simulink model "test"  (R2024a)
settings: Solver=VariableStepAuto  StartTime=0.0  StopTime=1000  RelTol=1e-3
undefined symbols (not defined in the file or in its folder): x
libraries: simulink x2
settings Model: Creator=b_ant  LastModifiedBy=b_ant

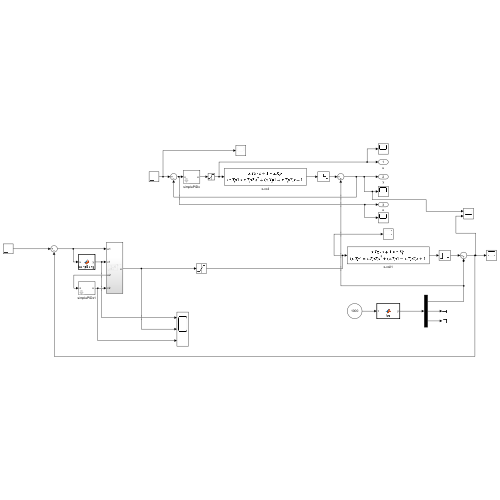
[thumbnail: Simulink's stored preview of the top-level diagram]
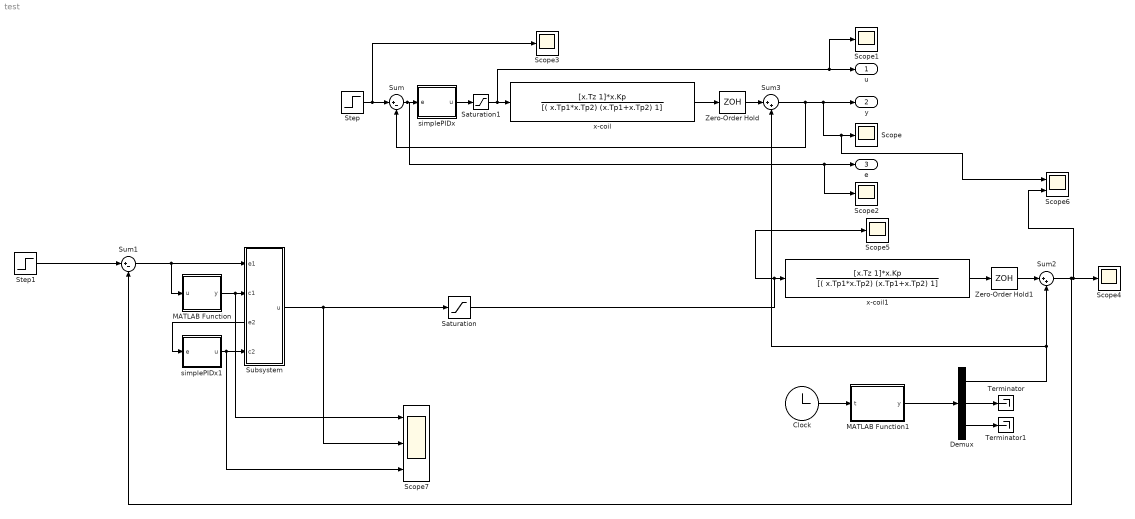
== system test ==
  Clock : Clock
  Demux : Demux  Outputs=3
  MATLAB Function : MATLAB Function  TreatAsAtomicUnit=on
  MATLAB Function1 : MATLAB Function  TreatAsAtomicUnit=on
  Saturation : Saturate  UpperLimit=15  LowerLimit=-15
  Saturation1 : Saturate  UpperLimit=15  LowerLimit=-15
  Scope{,1..5} (6 alike) : Scope
  Scope6 : Scope  NumInputPorts=2
  Scope7 : Scope  NumInputPorts=3
  Step : Step  Time=0.0001  SampleTime=0
  Step1 : Step  Time=0.0001  SampleTime=0
  Subsystem : Subsystem
      settings: PortSchema="{\"entries\":[{\"content\":{\"sides\":[{\"content\":{\"connectorIds\":[\"In1\",\"In2\",\"Out2\",\"In3\"]},\"type\":\"ConnectorPlacement.EquallySpacedRectSide\",\"uuid\":\"7068f7a8-39a5-4b81-9242-0ff684ad2d52\"},{\"content\":{\"connectorIds\":[\"Out1\"],\"side\":\"RIGHT\"},\"type\":\"ConnectorPlacement.EquallySpacedRectSide\",\"uuid\":\"6f619d2f-5996-4772-917a-a91f12c99af0\"},{\"content\":{\"side\":\"TOP\"},\"type\":\"ConnectorPlacement.EquallySpacedRectSide\",\"uuid\":\"a18f3392-cfd4-4b10-bccf-639e40fe0ff5\"}]},\"type\":\"ConnectorPlacement.EquallySpacedConnector\",\"uuid\":\"3030bedd-17ea-4c41-8905-7d24d55e9816\"}],\"packageUris\":[\"http://schema.mathworks.com/mf0/Connector/R2020b\"],\"version\":\"1.0\"}"
  Sum : Sum  Inputs=|+-
  Sum1 : Sum  Inputs=|+-
  Sum2 : Sum  Inputs=|++
  Sum3 : Sum  Inputs=|++
  Terminator : Terminator
  Terminator1 : Terminator
  Zero-Order Hold : ZeroOrderHold
  Zero-Order Hold1 : ZeroOrderHold
  simplePIDx : Subsystem  mask{Gain1=x.PID.Kd, Gain2=x.PID.Ki, Gain3=x.PID.Kp}
      mask prompts: Gain1 "kd:"; Gain2 "ki:"; Gain3 "kp:"
      mask TypeOptions Gain1: PID kd/Gain
      mask TypeOptions Gain2: PID ki/Gain
      mask TypeOptions Gain3: PID kp/Gain
  simplePIDx1 : Subsystem  mask{Gain1=x.PID.Kd, Gain2=x.PID.Ki, Gain3=x.PID.Kp}
      mask prompts: Gain1 "kd:"; Gain2 "ki:"; Gain3 "kp:"
      mask TypeOptions Gain1: PID kd/Gain
      mask TypeOptions Gain2: PID ki/Gain
      mask TypeOptions Gain3: PID kp/Gain
  x-coil : TransferFcn  Numerator=[x.Tz 1]*x.Kp  Denominator=[( x.Tp1*x.Tp2) (x.Tp1+x.Tp2) 1]
  x-coil1 : TransferFcn  Numerator=[x.Tz 1]*x.Kp  Denominator=[( x.Tp1*x.Tp2) (x.Tp1+x.Tp2) 1]
  u : Outport
  y : Outport  Port=2
  e : Outport  Port=3
  wires:
  x-coil/1 -> Zero-Order Hold/1
  simplePIDx/1(u) -> Saturation1/1
  Step/1 -> Scope3/1, Sum/1
  x-coil1/1 -> Zero-Order Hold1/1
  Step1/1 -> Sum1/1
  MATLAB Function1/1(y) -> Demux/1
  Clock/1 -> MATLAB Function1/1(t)
  Zero-Order Hold1/1 -> Sum2/1
  Sum2/1 -> Scope4/1, Scope6/2, Sum1/2
  Demux/1 -> Sum3/2, Sum2/2
  Demux/2 -> Terminator/1
  Demux/3 -> Terminator1/1
  Saturation/1 -> Scope5/1, x-coil1/1
  Zero-Order Hold/1 -> Sum3/1
  Sum3/1 -> Sum/2, Scope6/1, Scope/1, y/1
  Sum/1 -> Scope2/1, e/1, simplePIDx/1(e)
  Saturation1/1 -> Scope1/1, u/1, x-coil/1
  Sum1/1 -> MATLAB Function/1(u), Subsystem/1(e1)
  Subsystem/1(u) -> Scope7/2, Saturation/1
  simplePIDx1/1(u) -> Scope7/3, Subsystem/3(c2)
  Subsystem/2(e2) -> simplePIDx1/1(e)
  MATLAB Function/1(y) -> Scope7/1, Subsystem/2(c1)

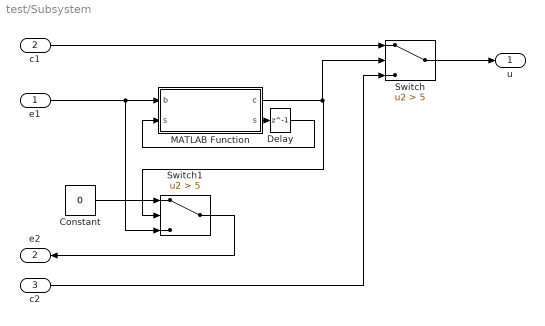
== system test/Subsystem ==
  e1 : Inport
  c1 : Inport  Port=2
  c2 : Inport  Port=3
  Constant : Constant  Value=0
  Delay : Delay  DelayLength=1
  MATLAB Function : MATLAB Function  TreatAsAtomicUnit=on
  Switch : Switch  Criteria=u2 > Threshold  Threshold=5  SaturateOnIntegerOverflow=off  InputSameDT=off
  Switch1 : Switch  Criteria=u2 > Threshold  Threshold=5  SaturateOnIntegerOverflow=off  InputSameDT=off
  u : Outport
  e2 : Outport  Port=2
  wires:
  e1/1 -> Switch1/3, MATLAB Function/1(b)
  MATLAB Function/2(s) -> Delay/1
  MATLAB Function/1(c) -> Switch/2, Switch1/2
  Switch1/1 -> e2/1
  Constant/1 -> Switch1/1
  c1/1 -> Switch/1
  Delay/1 -> MATLAB Function/2("s ")
  Switch/1 -> u/1
  c2/1 -> Switch/3

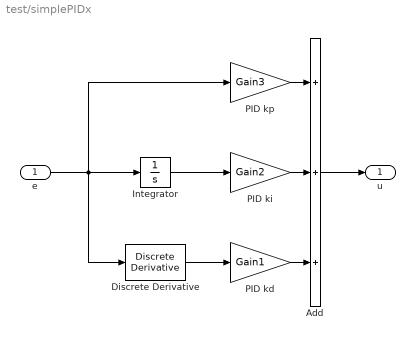
== system test/simplePIDx ==
  e : Inport
  Add : Sum  Inputs=+++
  Discrete Derivative : simulink/Discrete/Discrete Derivative  gainval=1.0  ICPrevScaledInput=0.0  OutMin=[]  OutMax=[]  OutDataType=fixdt(1, 16)  OutScaling=2^-10  DoSatur=off
  Integrator : Integrator
  PID kd : Gain  Gain=Gain1
  PID ki : Gain  Gain=Gain2
  PID kp : Gain  Gain=Gain3
  u : Outport
  wires:
  Discrete Derivative/1 -> PID kd/1
  Add/1 -> u/1
  e/1 -> PID kp/1, Integrator/1, Discrete Derivative/1
  Integrator/1 -> PID ki/1
  PID ki/1 -> Add/2
  PID kd/1 -> Add/3
  PID kp/1 -> Add/1

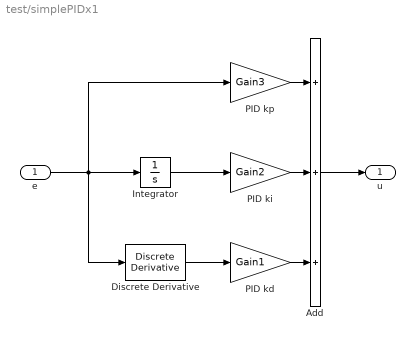
== system test/simplePIDx1 ==
  e : Inport
  Add : Sum  Inputs=+++
  Discrete Derivative : simulink/Discrete/Discrete Derivative  gainval=1.0  ICPrevScaledInput=0.0  OutMin=[]  OutMax=[]  OutDataType=fixdt(1, 16)  OutScaling=2^-10  DoSatur=off
  Integrator : Integrator
  PID kd : Gain  Gain=Gain1
  PID ki : Gain  Gain=Gain2
  PID kp : Gain  Gain=Gain3
  u : Outport
  wires:
  Discrete Derivative/1 -> PID kd/1
  Add/1 -> u/1
  e/1 -> PID kp/1, Integrator/1, Discrete Derivative/1
  Integrator/1 -> PID ki/1
  PID ki/1 -> Add/2
  PID kd/1 -> Add/3
  PID kp/1 -> Add/1

== matlab function test/Subsystem/MATLAB Function ==
  data: b input; c output; s input; s output
function [c,s] = selector(b,s)
if(and(or(b >= 100, b <= -100),s==0))
    c = 10;
else
    c = 0;
    s = 1;
end

== matlab function test/MATLAB Function ==
  data: u input; y output
function y = bangBang(u)
    y = 15*sign(u);
end

== matlab function test/MATLAB Function1 ==
  data: t input; y output
function y = fcn(t)
y= [2.522*sin(2*pi*4.788E-3*t)+3.249E04;
   -5.174*sin(2*pi*7.481E-3*t)-2.265E04;
    3.359*sin(2*pi*8.378E-3*t)+3.655E04];
end
